simulink model "distMoment"  (R2023b)
settings: Solver=VariableStepAuto  StartTime=0.0  StopTime=10.0  RelTol=1e-3
undefined symbols (not defined in the file): I_sim, magnitude
libraries: matrix_library x2
settings Model: Creator=kristopherriordan  LastModifiedBy=kristopherriordan

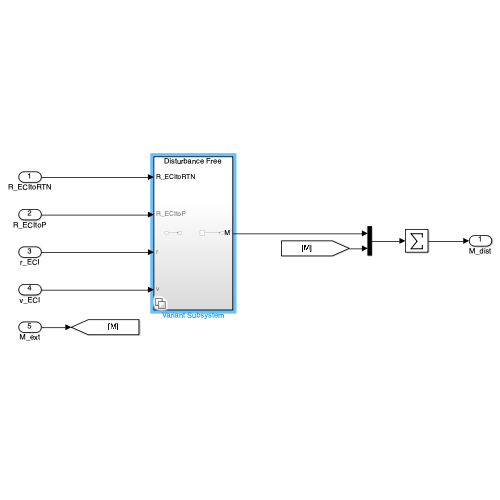
[thumbnail: Simulink's stored preview of the top-level diagram]
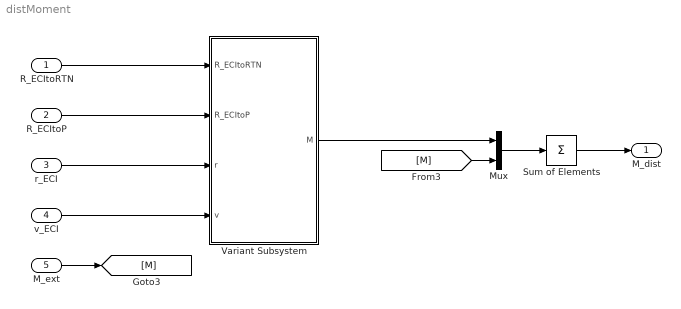
== system distMoment ==
  R_ECItoRTN : Inport
  R_ECItoP : Inport  Port=2
  r_ECI : Inport  Port=3
  v_ECI : Inport  Port=4
  M_ext : Inport  Port=5
  Mux : Mux  Inputs=2
  Sum of Elements : Sum  Inputs=+
  Variant Subsystem : Subsystem  Variant=on
  M_dist : Outport
  wires:
  M_ext/1 -> [M]
  R_ECItoRTN/1 -> Variant Subsystem/1(R_ECItoRTN)
  r_ECI/1 -> Variant Subsystem/3(r)
  v_ECI/1 -> Variant Subsystem/4(v)
  Mux/1 -> Sum of Elements/1
  Variant Subsystem/1(M) -> Mux/1
  [M] -> Mux/2
  Sum of Elements/1 -> M_dist/1
  R_ECItoP/1 -> Variant Subsystem/2(R_ECItoP)

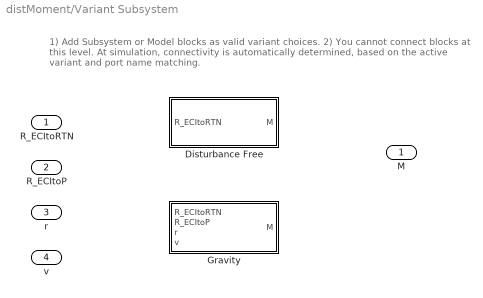
== system distMoment/Variant Subsystem ==
  note: 1) Add Subsystem or Model blocks as valid variant choices.
      | 2) You cannot connect blocks at this level. At simulation, connectivity is automatically
      | determined, based on the active variant and port name matching.
  R_ECItoRTN : Inport
  R_ECItoP : Inport  Port=2
  r : Inport  Port=3
  v : Inport  Port=4
  Disturbance Free : Subsystem  VariantControl=true
  Gravity : Subsystem  VariantControl=false
  M : Outport

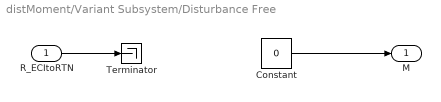
== system distMoment/Variant Subsystem/Disturbance Free ==
  R_ECItoRTN : Inport
  Constant : Constant  Value=0
  Terminator : Terminator
  M : Outport
  wires:
  Constant/1 -> M/1
  R_ECItoRTN/1 -> Terminator/1

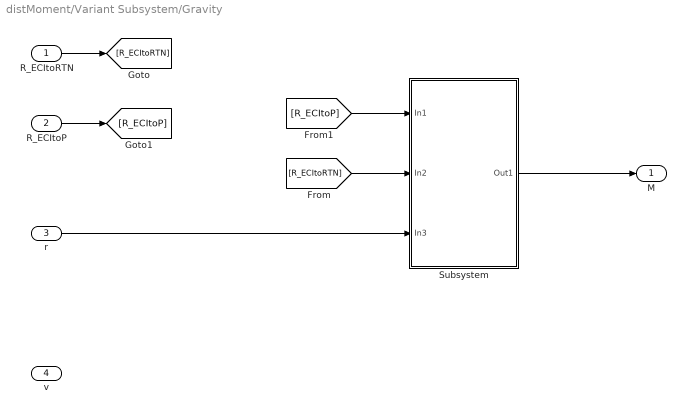
== system distMoment/Variant Subsystem/Gravity ==
  R_ECItoRTN : Inport
  R_ECItoP : Inport  Port=2
  r : Inport  Port=3
  v : Inport  Port=4
  Subsystem : Subsystem
  M : Outport
  wires:
  R_ECItoRTN/1 -> [R_ECItoRTN]
  R_ECItoP/1 -> [R_ECItoP]
  [R_ECItoP] -> Subsystem/1(In1)
  [R_ECItoRTN] -> Subsystem/2(In2)
  r/1 -> Subsystem/3(In3)
  Subsystem/1(Out1) -> M/1

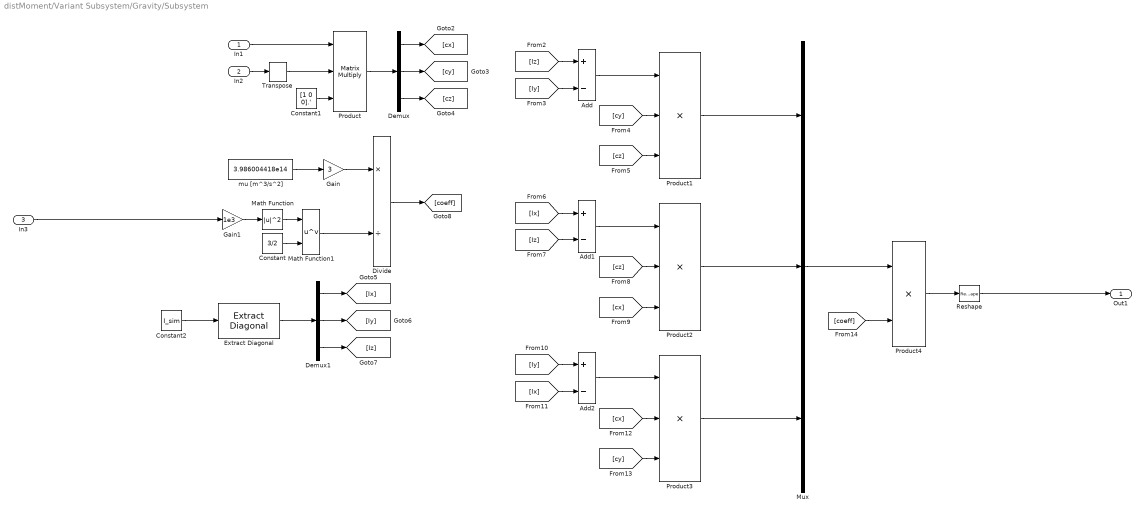
== system distMoment/Variant Subsystem/Gravity/Subsystem ==
  In1 : Inport
  In2 : Inport  Port=2
  In3 : Inport  Port=3
  Add : Sum  Inputs=+-
  Add1 : Sum  Inputs=+-
  Add2 : Sum  Inputs=+-
  Constant : Constant  Value=3/2
  Constant1 : Constant  Value=[1 0 0].'  VectorParams1D=off
  Constant2 : Constant  Value=I_sim
  Demux : Demux  Outputs=3
  Demux1 : Demux  Outputs=3
  Divide : Product  Inputs=*/
  Extract Diagonal : matrix_library/Extract Diagonal
      settings: LibrarySourceBlock=|
      | simulink/Matrix
      | Operations/Extract Diagonal
  Gain : Gain  Gain=3
  Gain1 : Gain  Gain=1e3
  Math Function : Math  Operator=magnitude^2
  Math Function1 : Math  Operator=pow
  Mux : Mux  Inputs=3
  Product : Product  Inputs=***  Multiplication=Matrix(*)
  Product1 : Product  Inputs=***
  Product2 : Product  Inputs=***
  Product3 : Product  Inputs=***
  Product4 : Product
  Reshape : Reshape  OutputDimensionality=Column vector (2-D)
  Transpose : matrix_library/Transpose
  mu [m^3/s^2] : Constant  Value=3.986004418e14
  Out1 : Outport
  wires:
  [cx] -> Product2/3
  Demux/1 -> [cx]
  Demux1/2 -> [Iy]
  [Iy] -> Add/2
  Mux/1 -> Product4/1
  Product4/1 -> Reshape/1
  Product1/1 -> Mux/1
  Demux1/1 -> [Ix]
  Product2/1 -> Mux/2
  In2/1 -> Transpose/1
  Math Function1/1 -> Divide/2
  Constant/1 -> Math Function1/2
  Gain/1 -> Divide/1
  Add1/1 -> Product2/1
  [cx] -> Product3/2
  [cy] -> Product1/2
  [cy] -> Product3/3
  Reshape/1 -> Out1/1
  [Iz] -> Add/1
  Product3/1 -> Mux/3
  [Iy] -> Add2/1
  [Ix] -> Add2/2
  Transpose/1 -> Product/2
  Demux/2 -> [cy]
  [Iz] -> Add1/2
  In1/1 -> Product/1
  Extract Diagonal/1 -> Demux1/1
  [cz] -> Product1/3
  Divide/1 -> [coeff]
  Demux1/3 -> [Iz]
  Add/1 -> Product1/1
  [coeff] -> Product4/2
  Demux/3 -> [cz]
  [Ix] -> Add1/1
  Constant1/1 -> Product/3
  [cz] -> Product2/2
  In3/1 -> Gain1/1
  Gain1/1 -> Math Function/1
  Add2/1 -> Product3/1
  Math Function/1 -> Math Function1/1
  mu [m^3/s^2]/1 -> Gain/1
  Product/1 -> Demux/1
  Constant2/1 -> Extract Diagonal/1
